simulink model "Blending_Challenge"  (Simulink 10.0)
settings: Solver=ode45  StartTime=0.0  StopTime=46  RelTol=1e-3  EnableMultiTasking=on
InitFcn:
  | FG_Initialize_Data
StopFcn:
  | FG_Cleanup_Data
undefined symbols (not defined in the file): DiscIntNeverNeededParam, Feed_Gas_Metering_Bias, FG_InitCond, FG_Scenario, Fuel_Gas_Demand_Seed, Fuel_Gas_HHV_Seed, Fuel_Gas_WI_Seed
libraries: simulink x1
settings Model: FPTRunName=Active  Creator=larry  LastModifiedBy=bhisma
settings DataIOCC: SignalLoggingSaveFormat=ModelDataLogs  SaveOutput=off  SignalLogging=off  DSMLogging=off  SaveTime=off  ReturnWorkspaceOutputsName=simOut
settings OptimizationCC: ExpressionDepthLimit=2147483647
settings DebuggingCC: FcnCallInpInsideContextMsg=warning  StateNameClashWarn=warning
settings GRTTargetCC: GeneratePreprocessorConditionals=Disable all
settings ConfigComp: CovExternalEMLEnable=off

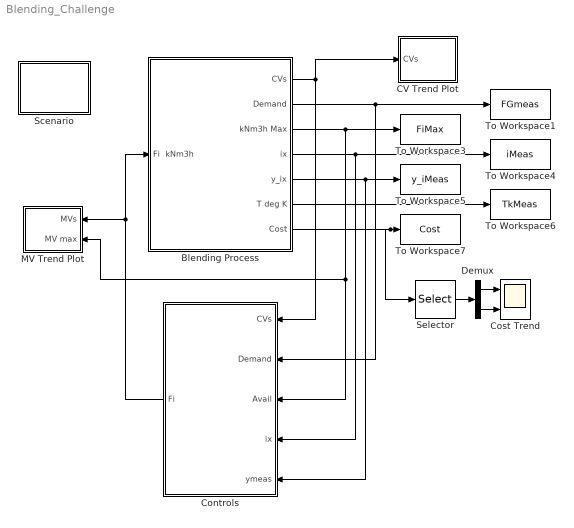
== system Blending_Challenge ==
  Blending Process : Subsystem
  CV Trend Plot : Subsystem
  Controls : Subsystem
  Cost Trend : Scope  NumInputPorts=2
  Demux : Demux  Outputs=2
  MV Trend Plot : Subsystem
  Scenario : Subsystem  mask{FG_Scenario=1}
      mask prompts: FG_Scenario "Enter case to be run"
      mask Display: fprintf('Case = %i', FG_Scenario)
  Selector : Selector  InputPortWidth=3  IndexOptions=Index vector (dialog)  Indices=[1 3]  OutputSizes=1
  To Workspace1 : ToWorkspace  VariableName=FGmeas  SampleTime=-1
  To Workspace3 : ToWorkspace  VariableName=FiMax  SampleTime=-1
  To Workspace4 : ToWorkspace  VariableName=iMeas  SampleTime=-1
  To Workspace5 : ToWorkspace  VariableName=y_iMeas  SampleTime=-1
  To Workspace6 : ToWorkspace  VariableName=TkMeas  SampleTime=-1
  To Workspace7 : ToWorkspace  VariableName=Cost  SampleTime=-1
  wires:
  Blending Process/3(kNm3h Max) -> To Workspace3/1, Controls/3(Avail), MV Trend Plot/2(MV max)
  Blending Process/4(ix) -> To Workspace4/1, Controls/4(ix)
  Blending Process/2(Demand) -> To Workspace1/1, Controls/2(Demand)
  Blending Process/5(y_ix) -> To Workspace5/1, Controls/5(ymeas)
  Blending Process/6(T deg K) -> To Workspace6/1
  Controls/1(Fi) -> Blending Process/1(Fi  kNm3h), MV Trend Plot/1(MVs)
  Blending Process/1(CVs) -> CV Trend Plot/1(CVs), Controls/1(CVs)
  Blending Process/7(Cost) -> To Workspace7/1, Selector/1
  Demux/1 -> Cost Trend/1
  Demux/2 -> Cost Trend/2
  Selector/1 -> Demux/1

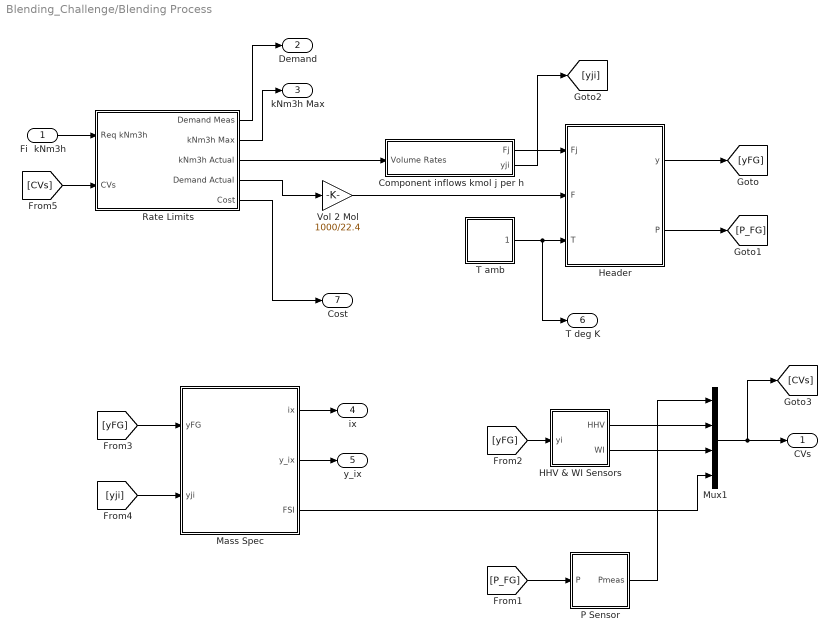
== system Blending_Challenge/Blending Process ==
  Fi  kNm3h : Inport
  Component inflows kmol j per h : Subsystem
  HHV & WI Sensors : Subsystem  mask{HHVi=[37.78, 126.5, 12.10, 0, 11.97, 0]}
      mask prompts: HHVi "HHV of chemicals"
      mask init:
      | Nc = length(HHVi);
  Header : Subsystem  mask{R=8.314, V=100, Z=1.006, Ni0=[14.7311, 1.0107, 47.8064, 4.5173, 9.6596, 5.9680]}
      mask prompts: R "R (gas law constant)"; V "Header Volume"; Z "Z (real gas correction factor)"; Ni0 "Initial state (moles of each chem)"
      mask init:
      | Nc = length(Ni0);
  Mass Spec : Subsystem
  Mux1 : Mux
  P Sensor : Subsystem
  Rate Limits : Subsystem
  T amb : Subsystem
  Vol 2 Mol : Gain  Gain=1000/22.4
  CVs : Outport  SampleTime=20/3600
  Demand : Outport  Port=2  SampleTime=20/3600
  kNm3h Max : Outport  Port=3  SampleTime=20/3600
  ix : Outport  Port=4  SampleTime=20/3600
  y_ix : Outport  Port=5  SampleTime=20/3600
  T deg K : Outport  Port=6  SampleTime=20/3600
  Cost : Outport  Port=7  SampleTime=20/3600
  wires:
  Mux1/1 -> CVs/1, [CVs]
  Component inflows kmol j per h/1(Fj) -> Header/1(Fj)
  T amb/1(T deg K) -> Header/3(T), T deg K/1
  Fi  kNm3h/1 -> Rate Limits/1(Req kNm3h)
  Rate Limits/1(Demand Meas) -> Demand/1
  Rate Limits/2(kNm3h Max) -> kNm3h Max/1
  Rate Limits/3(kNm3h Actual) -> Component inflows kmol j per h/1(Volume Rates)
  Header/1(y) -> [yFG]
  Header/2(P) -> [P_FG]
  [P_FG] -> P Sensor/1(P)
  [yFG] -> HHV & WI Sensors/1(yi)
  Mass Spec/1(ix) -> ix/1
  Mass Spec/2(y_ix) -> y_ix/1
  [yFG] -> Mass Spec/1(yFG)
  Vol 2 Mol/1 -> Header/2(F)
  Rate Limits/4(Demand Actual) -> Vol 2 Mol/1
  P Sensor/1(Pmeas) -> Mux1/1
  HHV & WI Sensors/1(HHV) -> Mux1/2
  Mass Spec/3(FSI) -> Mux1/4
  HHV & WI Sensors/2(WI) -> Mux1/3
  Component inflows kmol j per h/2(yji) -> [yji]
  [yji] -> Mass Spec/2(yji)
  Rate Limits/5(Cost) -> Cost/1
  [CVs] -> Rate Limits/2(CVs)

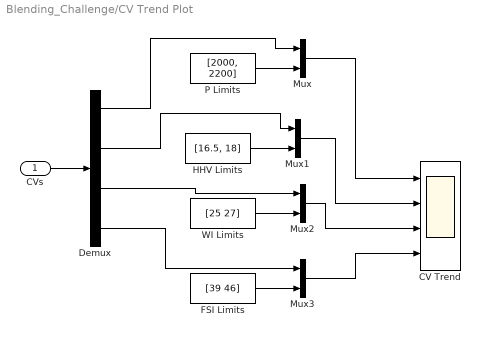
== system Blending_Challenge/CV Trend Plot ==
  CVs : Inport
  CV Trend : Scope  NumInputPorts=4
  Demux : Demux
  FSI Limits : Constant  Value=[39 46]
  HHV Limits : Constant  Value=[16.5, 18]
  Mux{,1..3} (4 alike) : Mux  Inputs=2
  P Limits : Constant  Value=[2000, 2200]
  WI Limits : Constant  Value=[25 27]
  wires:
  CVs/1 -> Demux/1
  P Limits/1 -> Mux/2
  Demux/1 -> Mux/1
  Mux/1 -> CV Trend/1
  HHV Limits/1 -> Mux1/2
  Demux/2 -> Mux1/1
  Mux1/1 -> CV Trend/2
  WI Limits/1 -> Mux2/2
  Demux/3 -> Mux2/1
  Mux2/1 -> CV Trend/3
  Mux3/1 -> CV Trend/4
  FSI Limits/1 -> Mux3/2
  Demux/4 -> Mux3/1

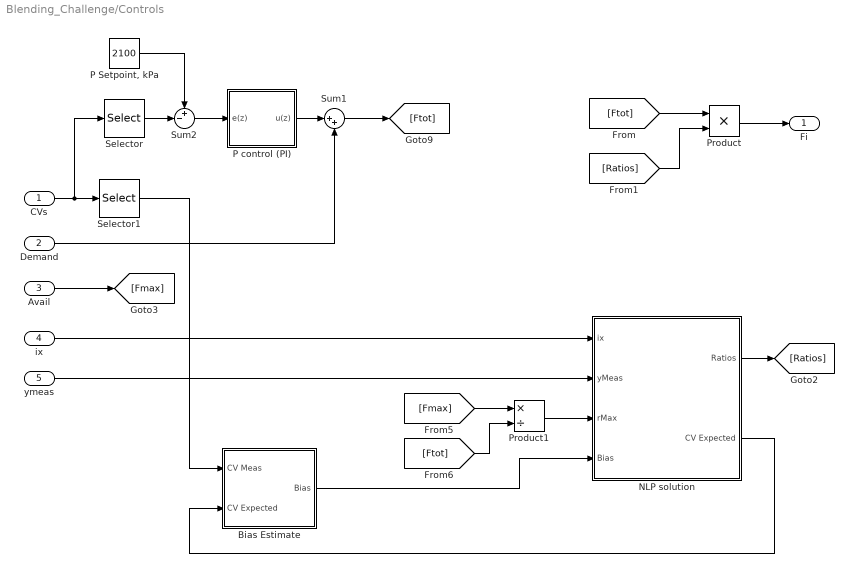
== system Blending_Challenge/Controls ==
  CVs : Inport
  Demand : Inport  Port=2
  Avail : Inport  Port=3
  ix : Inport  Port=4
  ymeas : Inport  Port=5
  Bias Estimate : Subsystem
  NLP solution : Subsystem
  "P Setpoint, kPa" : Constant  Value=2100
  P control (PI) : Subsystem
  Product : Product  RndMeth=Zero
  Product1 : Product  Inputs=*/  RndMeth=Zero
  Selector : Selector  InputPortWidth=4  IndexOptions=Index vector (dialog)  Indices=1  OutputSizes=1
  Selector1 : Selector  InputPortWidth=4  IndexOptions=Index vector (dialog)  Indices=2:4  OutputSizes=1
  Sum1 : Sum  Inputs=|++
  Sum2 : Sum  Inputs=+-|
  Fi : Outport
  wires:
  Demand/1 -> Sum1/2
  "P Setpoint, kPa"/1 -> Sum2/1
  Sum2/1 -> P control (PI)/1(e(z))
  P control (PI)/1(u(z)) -> Sum1/1
  Avail/1 -> [Fmax]
  Sum1/1 -> [Ftot]
  [Ftot] -> Product/1
  [Ratios] -> Product/2
  Product/1 -> Fi/1
  NLP solution/1(Ratios) -> [Ratios]
  [Fmax] -> Product1/1
  [Ftot] -> Product1/2
  Selector/1 -> Sum2/2
  CVs/1 -> Selector/1, Selector1/1
  Selector1/1 -> Bias Estimate/1(CV Meas)
  ix/1 -> NLP solution/1(ix)
  ymeas/1 -> NLP solution/2(yMeas)
  Product1/1 -> NLP solution/3(rMax)
  Bias Estimate/1(Bias) -> NLP solution/4(Bias)
  NLP solution/2(CV Expected) -> Bias Estimate/2(CV Expected)

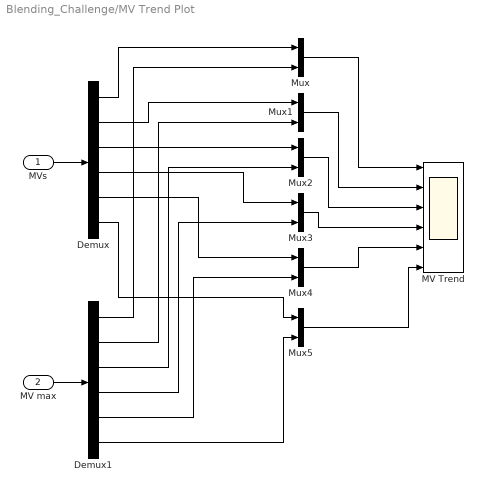
== system Blending_Challenge/MV Trend Plot ==
  MVs : Inport
  MV max : Inport  Port=2
  Demux : Demux  Outputs=6
  Demux1 : Demux  Outputs=6
  MV Trend : Scope  NumInputPorts=6
  Mux{,1..5} (6 alike) : Mux  Inputs=2
  wires:
  Demux/4 -> Mux3/1
  Mux3/1 -> MV Trend/4
  Mux2/1 -> MV Trend/3
  Demux/3 -> Mux2/1
  Mux1/1 -> MV Trend/2
  Demux/2 -> Mux1/1
  Mux/1 -> MV Trend/1
  Demux/1 -> Mux/1
  Demux1/1 -> Mux/2
  MVs/1 -> Demux/1
  MV max/1 -> Demux1/1
  Demux1/2 -> Mux1/2
  Demux1/3 -> Mux2/2
  Demux1/4 -> Mux3/2
  Mux4/1 -> MV Trend/5
  Demux/5 -> Mux4/1
  Demux1/5 -> Mux4/2
  Demux/6 -> Mux5/1
  Demux1/6 -> Mux5/2
  Mux5/1 -> MV Trend/6

== system Blending_Challenge/Scenario ==

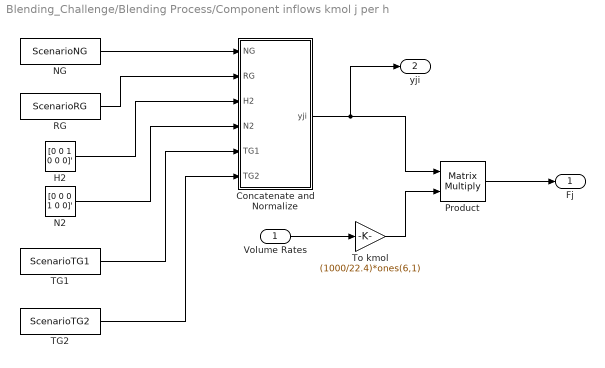
== system Blending_Challenge/Blending Process/Component inflows kmol j per h ==
  Volume Rates : Inport
  Concatenate and Normalize : MATLAB Function  TreatAsAtomicUnit=on
  H2 : Constant  Value=[0 0 1 0 0 0]'  VectorParams1D=off  SampleTime=20/3600
  N2 : Constant  Value=[0 0 0 1 0 0]'  VectorParams1D=off  SampleTime=20/3600
  NG : FromFile  FileName=ScenarioNG  SampleTime=20/3600  ExtrapolationBeforeFirstDataPoint=Hold first value  ExtrapolationAfterLastDataPoint=Hold last value
  Product : Product  Multiplication=Matrix(*)  RndMeth=Zero
  RG : FromFile  FileName=ScenarioRG  SampleTime=20/3600  ExtrapolationBeforeFirstDataPoint=Hold first value  ExtrapolationAfterLastDataPoint=Hold last value
  TG1 : FromFile  FileName=ScenarioTG1  SampleTime=20/3600  ExtrapolationBeforeFirstDataPoint=Hold first value  ExtrapolationAfterLastDataPoint=Hold last value
  TG2 : FromFile  FileName=ScenarioTG2  SampleTime=20/3600  ExtrapolationBeforeFirstDataPoint=Hold first value  ExtrapolationAfterLastDataPoint=Hold last value
  To kmol : Gain  Gain=(1000/22.4)*ones(6,1)
  Fj : Outport
  yji : Outport  Port=2
  wires:
  Product/1 -> Fj/1
  Volume Rates/1 -> To kmol/1
  To kmol/1 -> Product/2
  Concatenate and Normalize/1(yji) -> yji/1, Product/1
  NG/1 -> Concatenate and Normalize/1(NG)
  RG/1 -> Concatenate and Normalize/2(RG)
  H2/1 -> Concatenate and Normalize/3(H2)
  N2/1 -> Concatenate and Normalize/4(N2)
  TG1/1 -> Concatenate and Normalize/5(TG1)
  TG2/1 -> Concatenate and Normalize/6(TG2)

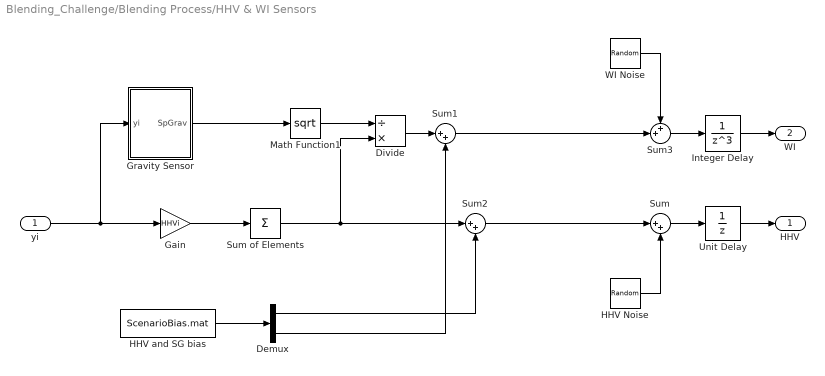
== system Blending_Challenge/Blending Process/HHV & WI Sensors ==
  yi : Inport  PortDimensions=Nc  SampleTime=20/3600
  Demux : Demux  Outputs=2
  Divide : Product  Inputs=/*
  Gain : Gain  Gain=HHVi
  Gravity Sensor : Subsystem  mask{MWTi=[16.04, 58.12, 2.016, 28.02, 28.01, 44.01], MWTair=28.8}
      mask prompts: MWTi "MWT of chemicals"; MWTair "MWT of standard gas"
      mask init:
      | Nc = length(MWTi);
  HHV Noise : RandomNumber  Variance=0.0049  Seed=Fuel_Gas_HHV_Seed(FG_Scenario)  SampleTime=20/3600
  HHV and SG bias : FromFile  FileName=ScenarioBias.mat  SampleTime=20/3600  ExtrapolationBeforeFirstDataPoint=Hold first value  ExtrapolationAfterLastDataPoint=Hold last value
  Integer Delay : DiscreteTransferFcn  Numerator=1  Denominator=[1 0 0 0]  InitialStates=25  SampleTime=20/3600
  Math Function1 : Math  Operator=sqrt  SaturateOnIntegerOverflow=on
  Sum : Sum  Inputs=|++
  Sum of Elements : Sum  Inputs=+
  Sum1 : Sum  Inputs=|++
  Sum2 : Sum  Inputs=|++
  Sum3 : Sum  Inputs=++|
  Unit Delay : UnitDelay  InitialCondition=16.5  SampleTime=20/3600  HasFrameUpgradeWarning=on
  WI Noise : RandomNumber  Variance=0.0049  Seed=Fuel_Gas_WI_Seed(FG_Scenario)  SampleTime=20/3600
  HHV : Outport
  WI : Outport  Port=2
  wires:
  Gain/1 -> Sum of Elements/1
  HHV Noise/1 -> Sum/2
  yi/1 -> Gain/1, Gravity Sensor/1(yi)
  Gravity Sensor/1(SpGrav) -> Math Function1/1
  HHV and SG bias/1 -> Demux/1
  Sum/1 -> Unit Delay/1
  Unit Delay/1 -> HHV/1
  Integer Delay/1 -> WI/1
  Math Function1/1 -> Divide/1
  Sum of Elements/1 -> Divide/2, Sum2/1
  Sum2/1 -> Sum/1
  Demux/1 -> Sum2/2
  Divide/1 -> Sum1/1
  Demux/2 -> Sum1/2
  WI Noise/1 -> Sum3/1
  Sum3/1 -> Integer Delay/1
  Sum1/1 -> Sum3/2

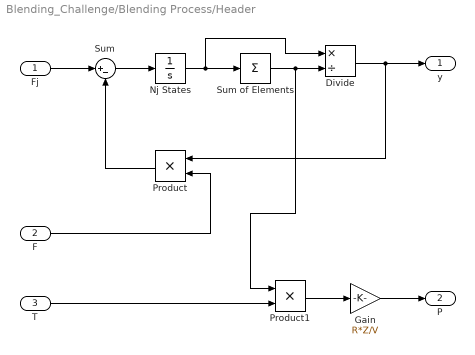
== system Blending_Challenge/Blending Process/Header ==
  Fj : Inport  PortDimensions=Nc
  F : Inport  Port=2  PortDimensions=1
  T : Inport  Port=3  PortDimensions=1
  Divide : Product  Inputs=*/
  Gain : Gain  Gain=R*Z/V
  Nj States : Integrator  InitialCondition=Ni0  LimitOutput=on  LowerSaturationLimit=0
  Product : Product  RndMeth=Zero
  Product1 : Product  RndMeth=Zero
  Sum : Sum  Inputs=|+-
  Sum of Elements : Sum  Inputs=+
  y : Outport
  P : Outport  Port=2
  wires:
  Nj States/1 -> Sum of Elements/1, Divide/1
  Sum/1 -> Nj States/1
  Sum of Elements/1 -> Divide/2, Product1/1
  Divide/1 -> y/1, Product/1
  Fj/1 -> Sum/1
  F/1 -> Product/2
  Product/1 -> Sum/2
  Gain/1 -> P/1
  Product1/1 -> Gain/1
  T/1 -> Product1/2

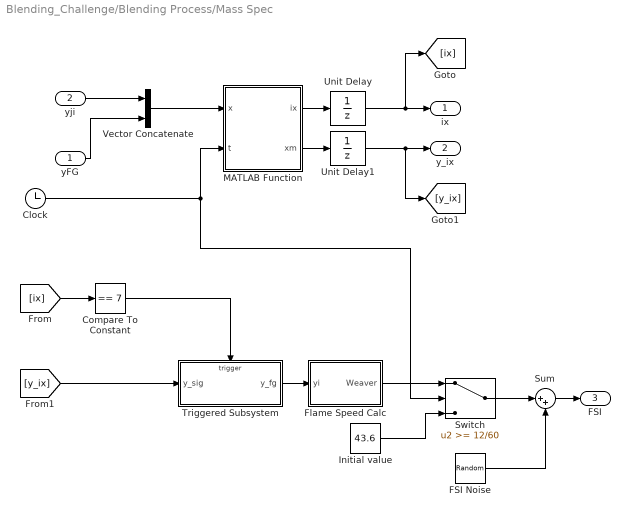
== system Blending_Challenge/Blending Process/Mass Spec ==
  yFG : Inport  SampleTime=20/3600
  yji : Inport  Port=2  SampleTime=20/3600
  Clock : Clock
  Compare To Constant : simulink/Logic and Bit Operations/Compare To Constant  relop===  const=7  OutDataTypeStr=uint8
  FSI Noise : RandomNumber  Variance=0.0049  Seed=Fuel_Gas_HHV_Seed(FG_Scenario)+4324  SampleTime=10/60
  Flame Speed Calc : Subsystem  mask{si=[148 514 339 0 61 0], Ai=[9.55 31 2.39 5 2.39 5]}
      mask prompts: si "si Factor"; Ai "Ai Factor"
      mask init:
      | Nc = length(si);
  Initial value : Constant  Value=43.6
  MATLAB Function : MATLAB Function  TreatAsAtomicUnit=on  SystemSampleTime=2/60
  Sum : Sum  Inputs=|++
  Switch : Switch  Threshold=12/60  SampleTime=2/60
  Triggered Subsystem : Subsystem  TreatAsAtomicUnit=on
  Unit Delay : UnitDelay  InitialCondition=7  SampleTime=2/60  HasFrameUpgradeWarning=on
  Unit Delay1 : UnitDelay  InitialCondition=[14.7311, 1.0107, 47.8064, 4.5173, 9.6596, 5.9680]'/83.6931  SampleTime=2/60  HasFrameUpgradeWarning=on
  Vector Concatenate : Concatenate  Mode=Multidimensional array  ConcatenateDimension=2
  ix : Outport  SampleTime=20/3600
  y_ix : Outport  Port=2  SampleTime=20/3600
  FSI : Outport  Port=3  SampleTime=20/3600
  wires:
  yFG/1 -> Vector Concatenate/2
  Clock/1 -> MATLAB Function/2(t), Switch/2
  Vector Concatenate/1 -> MATLAB Function/1(x)
  MATLAB Function/1(ix) -> Unit Delay/1
  MATLAB Function/2(xm) -> Unit Delay1/1
  [y_ix] -> Triggered Subsystem/1(y_sig)
  Triggered Subsystem/1(y_fg) -> Flame Speed Calc/1(yi)
  [ix] -> Compare To Constant/1
  Compare To Constant/1 -> Triggered Subsystem/Trigger
  Unit Delay1/1 -> y_ix/1, [y_ix]
  Unit Delay/1 -> ix/1, [ix]
  Flame Speed Calc/1(Weaver) -> Switch/1
  Initial value/1 -> Switch/3
  yji/1 -> Vector Concatenate/1
  FSI Noise/1 -> Sum/2
  Switch/1 -> Sum/1
  Sum/1 -> FSI/1

== system Blending_Challenge/Blending Process/P Sensor ==
  P : Inport  PortDimensions=1  SampleTime=20/3600
  Random Number : RandomNumber  Variance=25  Seed=4983498  SampleTime=20/3600
  Sum : Sum  Inputs=|++
  Pmeas : Outport
  wires:
  Sum/1 -> Pmeas/1
  P/1 -> Sum/1
  Random Number/1 -> Sum/2

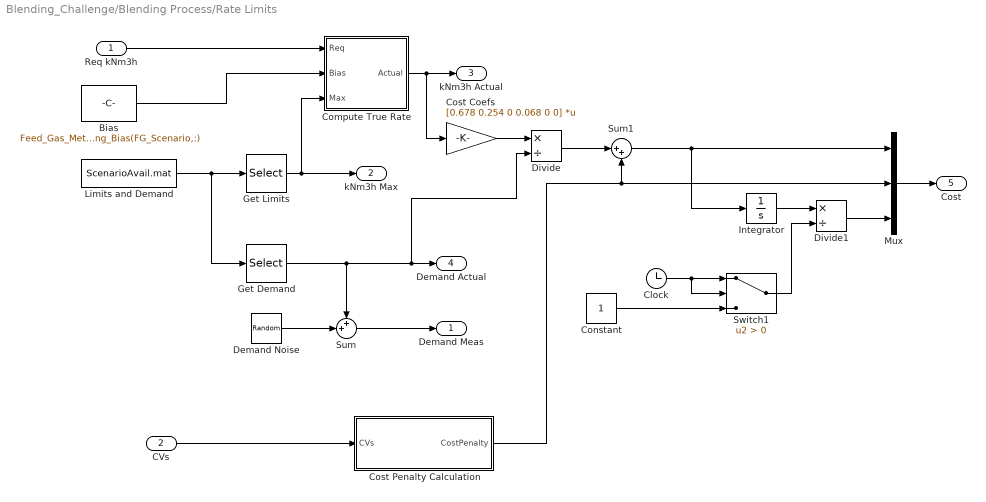
== system Blending_Challenge/Blending Process/Rate Limits ==
  Req kNm3h : Inport  OutMin=0  OutDataTypeStr=double  PortDimensions=6
  CVs : Inport  Port=2  OutMin=0  OutDataTypeStr=double  PortDimensions=4
  Bias : Constant  Value=Feed_Gas_Metering_Bias(FG_Scenario,:)
  Clock : Clock
  Compute True Rate : MATLAB Function  TreatAsAtomicUnit=on
  Constant : Constant
  Cost Coefs : Gain  Gain=[0.678 0.254 0 0.068 0 0]  Multiplication=Matrix(K*u)
  Cost Penalty Calculation : MATLAB Function  TreatAsAtomicUnit=on
  Demand Noise : RandomNumber  Variance=0.8  Seed=Fuel_Gas_Demand_Seed(FG_Scenario)  SampleTime=10/3600
  Divide : Product  Inputs=*/
  Divide1 : Product  Inputs=*/
  Get Demand : Selector  InputPortWidth=7  IndexOptions=Index vector (dialog)  Indices=7  OutputSizes=1
  Get Limits : Selector  InputPortWidth=7  IndexOptions=Index vector (dialog)  Indices=1:6  OutputSizes=1
  Integrator : Integrator
  Limits and Demand : FromFile  FileName=ScenarioAvail.mat  SampleTime=20/3600  ExtrapolationBeforeFirstDataPoint=Hold first value  ExtrapolationAfterLastDataPoint=Hold last value
  Mux : Mux  Inputs=3
  Sum : Sum  Inputs=++|
  Sum1 : Sum  Inputs=|++
  Switch1 : Switch  Criteria=u2 > Threshold
  Demand Meas : Outport  SampleTime=20/3600
  kNm3h Max : Outport  Port=2  SampleTime=20/3600
  kNm3h Actual : Outport  Port=3  SampleTime=20/3600
  Demand Actual : Outport  Port=4  SampleTime=20/3600
  Cost : Outport  Port=5  SampleTime=20/3600
  wires:
  Limits and Demand/1 -> Get Limits/1, Get Demand/1
  Get Limits/1 -> kNm3h Max/1, Compute True Rate/3(Max)
  Get Demand/1 -> Sum/1, Demand Actual/1, Divide/2
  Demand Noise/1 -> Sum/2
  Sum/1 -> Demand Meas/1
  Mux/1 -> Cost/1
  Constant/1 -> Switch1/3
  Cost Coefs/1 -> Divide/1
  Integrator/1 -> Divide1/1
  Switch1/1 -> Divide1/2
  Clock/1 -> Switch1/1, Switch1/2
  CVs/1 -> Cost Penalty Calculation/1(CVs)
  Divide/1 -> Sum1/1
  Cost Penalty Calculation/1(CostPenalty) -> Sum1/2, Mux/2
  Sum1/1 -> Mux/1, Integrator/1
  Req kNm3h/1 -> Compute True Rate/1(Req)
  Compute True Rate/1(Actual) -> kNm3h Actual/1, Cost Coefs/1
  Bias/1 -> Compute True Rate/2(Bias)
  Divide1/1 -> Mux/3

== system Blending_Challenge/Blending Process/T amb ==
  Constant : Constant  Value=293
  Sine Wave : Sin  Amplitude=10  Frequency=2*pi/24  SampleTime=20/3600
  Sum : Sum  Inputs=|++
  T deg K : Outport
  wires:
  Constant/1 -> Sum/1
  Sum/1 -> T deg K/1
  Sine Wave/1 -> Sum/2

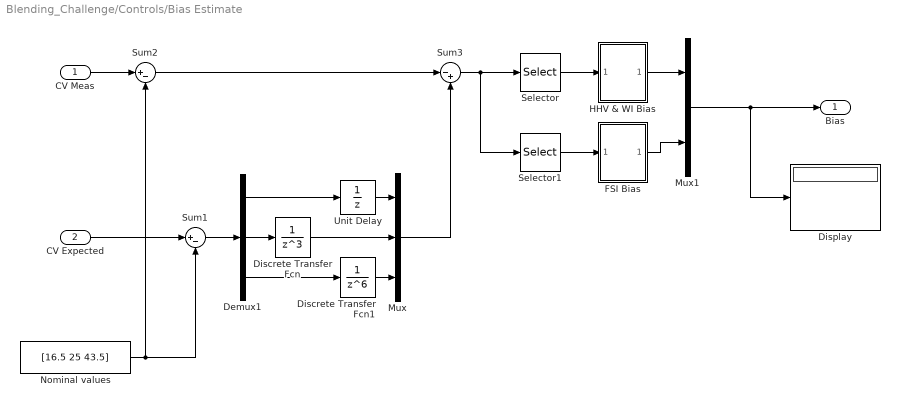
== system Blending_Challenge/Controls/Bias Estimate ==
  CV Meas : Inport  PortDimensions=3
  CV Expected : Inport  Port=2  PortDimensions=3
  Demux1 : Demux  Outputs=3
  Discrete Transfer Fcn : DiscreteTransferFcn  Denominator=[1 0 0 0]  SampleTime=20/3600
  Discrete Transfer Fcn1 : DiscreteTransferFcn  Denominator=[1 0 0 0 0 0 0]  SampleTime=20/3600
  Display : Display
  FSI Bias : Subsystem
  HHV & WI Bias : Subsystem
  Mux : Mux  Inputs=3
  Mux1 : Mux  Inputs=2
  Nominal values : Constant  Value=[16.5 25 43.5]
  Selector : Selector  InputPortWidth=3  IndexOptions=Index vector (dialog)  Indices=[1 2]  OutputSizes=1
  Selector1 : Selector  InputPortWidth=3  IndexOptions=Index vector (dialog)  Indices=[3]  OutputSizes=1
  Sum1 : Sum  Inputs=|+-
  Sum2 : Sum  Inputs=|+-
  Sum3 : Sum  Inputs=|-+
  Unit Delay : UnitDelay  SampleTime=20/3600  HasFrameUpgradeWarning=on
  Bias : Outport
  wires:
  CV Meas/1 -> Sum2/1
  CV Expected/1 -> Sum1/1
  Sum1/1 -> Demux1/1
  Nominal values/1 -> Sum1/2, Sum2/2
  Demux1/1 -> Unit Delay/1
  Demux1/2 -> Discrete Transfer Fcn/1
  Demux1/3 -> Discrete Transfer Fcn1/1
  Unit Delay/1 -> Mux/1
  Discrete Transfer Fcn/1 -> Mux/2
  Discrete Transfer Fcn1/1 -> Mux/3
  Sum2/1 -> Sum3/1
  Mux/1 -> Sum3/2
  Sum3/1 -> Selector/1, Selector1/1
  Selector/1 -> HHV & WI Bias/1(e(z))
  Selector1/1 -> FSI Bias/1(e(z))
  HHV & WI Bias/1(u(z)) -> Mux1/1
  FSI Bias/1(u(z)) -> Mux1/2
  Mux1/1 -> Bias/1, Display/1

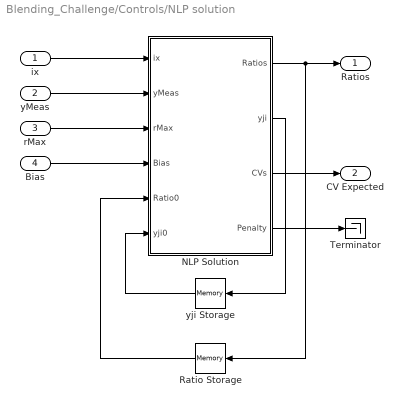
== system Blending_Challenge/Controls/NLP solution ==
  ix : Inport
  yMeas : Inport  Port=2
  rMax : Inport  Port=3
  Bias : Inport  Port=4
  NLP Solution : MATLAB Function  TreatAsAtomicUnit=on  SystemSampleTime=20/3600
  Ratio Storage : Memory  InitialCondition=[ 1.3983, 0, 4.2223, 0, 0, 24.3795]'/30
  Terminator : Terminator
  yji Storage : Memory  InitialCondition=FG_InitCond
  Ratios : Outport
  CV Expected : Outport  Port=2
  wires:
  ix/1 -> NLP Solution/1(ix)
  yMeas/1 -> NLP Solution/2(yMeas)
  Bias/1 -> NLP Solution/4(Bias)
  rMax/1 -> NLP Solution/3(rMax)
  NLP Solution/1(Ratios) -> Ratios/1, Ratio Storage/1
  NLP Solution/2(yji) -> yji Storage/1
  yji Storage/1 -> NLP Solution/6(yji0)
  Ratio Storage/1 -> NLP Solution/5(Ratio0)
  NLP Solution/3(CVs) -> CV Expected/1
  NLP Solution/4(Penalty) -> Terminator/1

== system Blending_Challenge/Controls/P control (PI) ==
  e(z) : Inport
  I mode : DiscreteIntegrator  gainval=1.8  SampleTime=20/3600  ICPrevOutput=DiscIntNeverNeededParam  ICPrevScaledInput=DiscIntNeverNeededParam
  P mode : Gain  Gain=0.08  SampleTime=20/3600
  Sum : Sum  Inputs=|++
  u(z) : Outport
  wires:
  Sum/1 -> u(z)/1
  P mode/1 -> Sum/1
  e(z)/1 -> P mode/1, I mode/1
  I mode/1 -> Sum/2

== system Blending_Challenge/Blending Process/HHV & WI Sensors/Gravity Sensor ==
  yi : Inport  PortDimensions=Nc
  Gain : Gain  Gain=MWTi
  Gain1 : Gain  Gain=1/MWTair
  Sum of Elements : Sum  Inputs=+
  SpGrav : Outport
  wires:
  yi/1 -> Gain/1
  Gain/1 -> Sum of Elements/1
  Sum of Elements/1 -> Gain1/1
  Gain1/1 -> SpGrav/1

== system Blending_Challenge/Blending Process/Mass Spec/Flame Speed Calc ==
  yi : Inport  PortDimensions=Nc
  Constant : Constant
  Divide : Product  Inputs=*/
  Gain : Gain  Gain=si
  Gain1 : Gain  Gain=Ai
  Sum : Sum  Inputs=|++
  Sum of Elements : Sum  Inputs=+
  Sum of Elements1 : Sum  Inputs=+
  Weaver : Outport
  wires:
  Sum of Elements/1 -> Divide/1
  Divide/1 -> Weaver/1
  Gain/1 -> Sum of Elements/1
  yi/1 -> Gain/1, Gain1/1
  Gain1/1 -> Sum of Elements1/1
  Sum of Elements1/1 -> Sum/1
  Constant/1 -> Sum/2
  Sum/1 -> Divide/2

== system Blending_Challenge/Blending Process/Mass Spec/Triggered Subsystem ==
  y_sig : Inport
  Trigger : TriggerPort  VariantControl=(inherit)
  y_fg : Outport
  wires:
  y_sig/1 -> y_fg/1

== system Blending_Challenge/Controls/Bias Estimate/FSI Bias ==
  e(z) : Inport  SampleTime=10/60
  Gain : Gain  Gain=0.2
  Sum2 : Sum  Inputs=|++
  Unit Delay : UnitDelay  SampleTime=-1  HasFrameUpgradeWarning=on
  u(z) : Outport
  wires:
  Unit Delay/1 -> Sum2/2
  Sum2/1 -> u(z)/1, Unit Delay/1
  e(z)/1 -> Gain/1
  Gain/1 -> Sum2/1

== system Blending_Challenge/Controls/Bias Estimate/HHV & WI Bias ==
  e(z) : Inport  SampleTime=20/3600
  Gain : Gain  Gain=0.2
  Sum2 : Sum  Inputs=|++
  Unit Delay : UnitDelay  SampleTime=-1  HasFrameUpgradeWarning=on
  u(z) : Outport
  wires:
  Unit Delay/1 -> Sum2/2
  Sum2/1 -> u(z)/1, Unit Delay/1
  Gain/1 -> Sum2/1
  e(z)/1 -> Gain/1

== matlab function Controls/NLP solution/NLP Solution ==
  data: Ratios output double size=6; ix input double size=1; yMeas input double size=6; rMax input double size=6; Bias input double size=3; Ratio0 input double size=6; yji output double size=[6,6]; yji0 input double size=[6,6]; CVs output double size=3; Penalty output double size=1
function [Ratios, yji, CVs, Penalty] = fcn(ix, yMeas, rMax, Bias, Ratio0, yji0)
%#codegen
coder.extrinsic('NLPcalc')

% Initialization
Ratios = Ratio0;
yji = yji0;
CVs = zeros(3,1);
Penalty = 0;

% If ix indicates a valid measurement, update the feed compositions
if ix >= 1 && ix <= 6
    yji(:,ix) = yMeas(:)/sum(yMeas);
end

% Nonlinear Programming solution
xGuess = [Ratio0(:); 0; 0; 0];
% NLP limits chosen to reduce likelihood of constraint violation
SafetyMargin = [0.25, 0.25, 0.5]';
Pmin = [16.5, 25, 39]' + SafetyMargin;  
Pmax = [18.0, 27, 46]' - SafetyMargin;
% The true process constraints are as follows:
% Pmin = [16.5,  25,  39]';
% Pmax = [18.0,  27,  46]';
[Ratios, CVs, Penalty] = NLPcalc(yji, rMax, Bias, 1, xGuess, Pmin, Pmax);

== matlab function Blending Process/Component inflows kmol j per h/Concatenate and Normalize ==
  data: NG input double size=6; yji output double; RG input double size=6; H2 input double size=6; N2 input double size=6; TG1 input double size=6; TG2 input double size=6
function yji = fcn(NG, RG, H2, N2, TG1, TG2)
%#codegen

NG = NG(:)/sum(NG);
RG = RG(:)/sum(RG);
H2 = H2(:)/sum(H2);
N2 = N2(:)/sum(N2);
TG1 = TG1(:)/sum(TG1);
TG2 = TG2(:)/sum(TG2);
yji = [NG RG H2 N2 TG1 TG2];

== matlab function Blending Process/Mass Spec/MATLAB Function ==
  data: x input double; ix output double; t input double; xm output double
function [ix, xm] = fcn(x, t)
%#codegen

Cycle = [1 2 5 6 7];    % Sampling sequence
ts = 2/60;              % Time per sample
BadProb = 1e-3*ones(1,7);
% Determine stream to be sampled now.
ix = Cycle(round(mod(round(t/ts), 5) + 1));
xm = x(:,ix);

% Possible bad/skipped measurement
if rand < BadProb(ix)
    % Bad
    ix = -ix;
    xm = zeros(size(xm));
end

== matlab function Blending Process/Rate Limits/Cost Penalty Calculation ==
  data: CVs input double size=4; CostPenalty output double size=1
function CostPenalty = fcn(CVs)
%#codegen

% Examine the CVs for constraint violations and penalize if found.

% CV bounds
CVmin = [2000 16.5 25 39]';
CVmax = [2200 18.0 27 46]';
% CV standard deviations
Sig = [5, 0.07*ones(1,3)]';
% Compute slack variables (>0 if constraint has been violated)
Eps = max(CVmin - CVs(:), 0) + max(CVs(:) - CVmax, 0) ;
% Compute penalty
CostPenalty = 0.02*sum((Eps ./ Sig).^2);

== matlab function Blending Process/Rate Limits/Compute True Rate ==
  data: Req input double size=6; Actual output double size=6; Bias input double size=6; Max input double size=6
function Actual = fcn(Req, Bias, Max)
%#codegen

Actual = zeros(6,1);
for i = 1:6
    if Req(i) > 0
        Actual(i) = max(0, min(Max(i), Req(i) + Bias(i)));
    end
end
